simulink model "projectsim2021"  (R2021b)
settings: Solver=VariableStepAuto  StartTime=0.0  StopTime=5  RelTol=1e-3
values from neighbouring files (symbols this model uses):
  n_max = [.1;.1]    [p3.m]
libraries: cstblocks x3, simulink x2
settings Model: Creator=wen  LastModifiedBy=dabner
settings DebuggingCC: ParameterPrecisionLossMsg=none  UnconnectedInputMsg=none  UnconnectedOutputMsg=none  UnconnectedLineMsg=none
settings ModelReferenceCC: EnableRefExpFcnMdlSchedulingChecks=off
settings RTWCC: DLArmComputeVersion=20.02.1

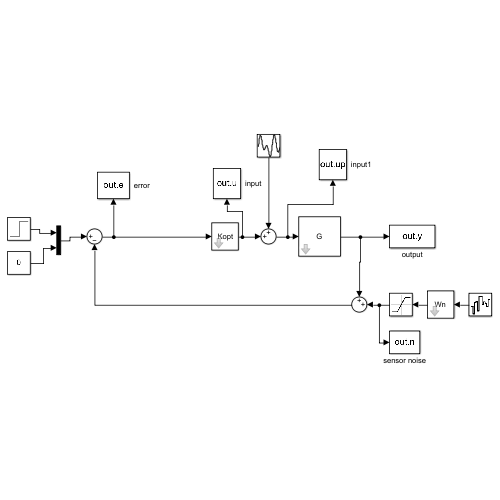
[thumbnail: Simulink's stored preview of the top-level diagram]
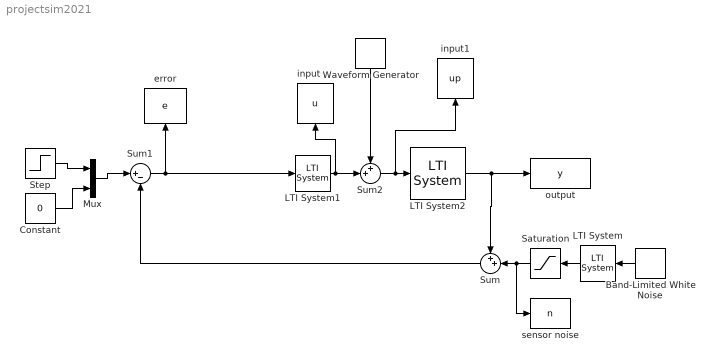
== system projectsim2021 ==
  Band-Limited White Noise : simulink/Sources/Band-Limited White Noise  Cov=n_power  Ts=0.1  seed=[23341]
  Constant : Constant  Value=0
  LTI System : cstblocks/LTI System  sys=Wn  IC=[]
  LTI System1 : cstblocks/LTI System  sys=Kopt  IC=[]
  LTI System2 : cstblocks/LTI System  sys=G  IC=[]
  Mux : Mux  Inputs=2
  Saturation : Saturate  UpperLimit=n_max  LowerLimit=-n_max
  Step : Step  SampleTime=0
  Sum : Sum  Inputs=++|
  Sum1 : Sum  Inputs=|+-
  Sum2 : Sum  Inputs=++|
  Waveform Generator : simulink/Sources/Waveform Generator  OutMin=[]  OutMax=[]  OutDataTypeStr=double  SelectedSignal=1  Signals=sin(a1,w1,0)#sin(a2,w2,pi/4)  BlockNames=MultiportSwitch_809c31518d074d9#MultiportSwitch_1a105935f6d147d  SampleTime=0.1
  error : ToWorkspace  VariableName=e  SampleTime=-1
  input : ToWorkspace  VariableName=u  SampleTime=-1
  input1 : ToWorkspace  VariableName=up  SampleTime=-1
  output : ToWorkspace  VariableName=y  SampleTime=-1
  sensor noise : ToWorkspace  VariableName=n  SampleTime=-1
  wires:
  LTI System2/1 -> Sum/1, output/1
  Sum/1 -> Sum1/2
  Sum2/1 -> input1/1, LTI System2/1
  Step/1 -> Mux/1
  Mux/1 -> Sum1/1
  Constant/1 -> Mux/2
  LTI System/1 -> Saturation/1
  Band-Limited White Noise/1 -> LTI System/1
  Saturation/1 -> sensor noise/1, Sum/2
  LTI System1/1 -> input/1, Sum2/2
  Sum1/1 -> LTI System1/1, error/1
  Waveform Generator/1 -> Sum2/1
